simulink model "mmr_air_alternat"  (R2019a)
settings: Solver=ode4  StartTime=0.0  StopTime=ta  RelTol=1e-1
values from neighbouring files (symbols this model uses):
  g = -9.81    [MMR.m]    (also in MMR_alfa0.m; MMR_alone.m; MMR_hop_zero.m = 9.81)
  Lcol = 0.70    (= 0.7)    [MMR.m]    (also in MMR_alone.m)
  Lhk = 0.28    [MMR.m]    (also in MMR_alfa0.m; MMR_alone.m; MMR_hop_zero.m)
  Lkf = 0.28    [MMR.m]    (also in MMR_alfa0.m; MMR_alone.m; MMR_hop_zero.m)
  m = 3    [MMR.m]    (also in MMR_alfa0.m; MMR_alone.m; MMR_hop_zero.m)
  M = 15    [MMR.m]    (also in MMR_alfa0.m; MMR_alone.m; MMR_hop_zero.m)
  vxfinal = vx( length(vx) )    [MMR.m]    (also in MMR_alfa0.m; MMR_alone.m)
  vxMfinal = vxM( length(vxM) )    [MMR.m]    (also in MMR_alfa0.m; MMR_alone.m)
  vyfinal = vy( length(vy) )    [MMR.m]    (also in MMR_alfa0.m; MMR_alone.m; MMR_hop_zero.m)
  vyMfinal = vyM( length(vyM) )    [MMR.m]    (also in MMR_alfa0.m; MMR_alone.m)
  xfinal = x( length(x) )    [MMR.m]    (also in MMR_alfa0.m; MMR_alone.m)
  xMfinal = xM( length(xM) )    [MMR.m]    (also in MMR_alfa0.m; MMR_alone.m)
  yfinal = y( length(y) )    [MMR.m]    (also in MMR_alfa0.m; MMR_alone.m; MMR_hop_zero.m)
  yMfinal = yM( length(yM) )    [MMR.m]    (also in MMR_alfa0.m; MMR_alone.m)
undefined symbols (not defined in the file or in its folder): magnitude
settings Model: Creator=Jesus  LastModifiedBy=Jesus

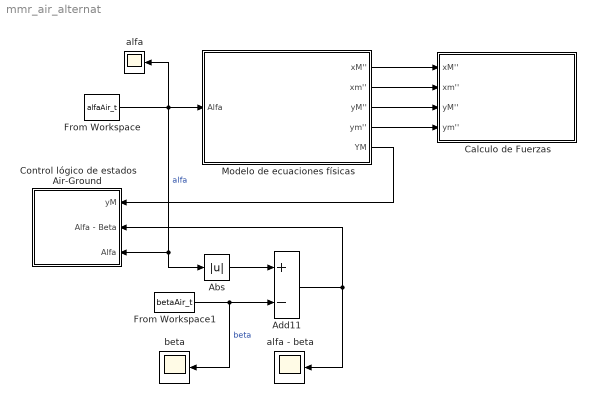
== system mmr_air_alternat ==
  Abs : Abs
  Add11 : Sum  Inputs=+-
  Calculo de Fuerzas : Subsystem
  Control lógico de estados Air-Ground : Subsystem
  From Workspace : FromWorkspace  VariableName=alfaAir_t  SampleTime=0
  From Workspace1 : FromWorkspace  VariableName=betaAir_t  SampleTime=0
  Modelo de ecuaciones físicas : Subsystem
  alfa : Scope
  alfa - beta : Scope
  beta : Scope
  wires:
  From Workspace/1 -> alfa/1, Control lógico de estados Air-Ground/3(Alfa), Abs/1, Modelo de ecuaciones físicas/1(Alfa)  "alfa"
  Add11/1 -> Control lógico de estados Air-Ground/2(Alfa - Beta), alfa - beta/1
  From Workspace1/1 -> beta/1, Add11/2  "beta"
  Modelo de ecuaciones físicas/1(xM'') -> Calculo de Fuerzas/1(xM'')
  Modelo de ecuaciones físicas/2(xm'') -> Calculo de Fuerzas/2(xm'')
  Modelo de ecuaciones físicas/3(yM'') -> Calculo de Fuerzas/3(yM'')
  Modelo de ecuaciones físicas/4(ym'') -> Calculo de Fuerzas/4(ym'')
  Modelo de ecuaciones físicas/5(YM) -> Control lógico de estados Air-Ground/1(yM)
  Abs/1 -> Add11/1

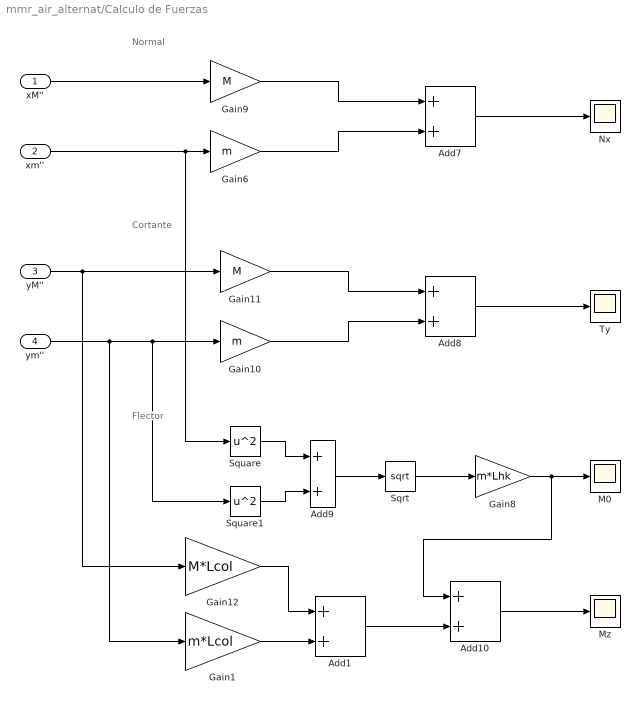
== system mmr_air_alternat/Calculo de Fuerzas ==
  note: Normal
  note: Cortante
  note: Flector
  xM'' : Inport
  xm'' : Inport  Port=2
  yM'' : Inport  Port=3
  ym'' : Inport  Port=4
  Add{1,7..10} (5 alike) : Sum
  Gain1 : Gain  Gain=m*Lcol
  Gain10 : Gain  Gain=m
  Gain11 : Gain  Gain=M
  Gain12 : Gain  Gain=M*Lcol
  Gain6 : Gain  Gain=m
  Gain8 : Gain  Gain=m*Lhk
  Gain9 : Gain  Gain=M
  M0 : Scope
  Mz : Scope
  Nx : Scope
  Sqrt : Sqrt  SaturateOnIntegerOverflow=on
  Square : Math  Operator=square  SaturateOnIntegerOverflow=on
  Square1 : Math  Operator=square  SaturateOnIntegerOverflow=on
  Ty : Scope
  wires:
  Gain10/1 -> Add8/2
  Sqrt/1 -> Gain8/1
  yM''/1 -> Gain11/1, Gain12/1
  ym''/1 -> Square1/1, Gain10/1, Gain1/1
  Square/1 -> Add9/1
  Add7/1 -> Nx/1
  Gain8/1 -> Add10/1, M0/1
  Gain6/1 -> Add7/2
  Gain11/1 -> Add8/1
  xm''/1 -> Square/1, Gain6/1
  Add9/1 -> Sqrt/1
  Add8/1 -> Ty/1
  Gain9/1 -> Add7/1
  Square1/1 -> Add9/2
  Add10/1 -> Mz/1
  xM''/1 -> Gain9/1
  Add1/1 -> Add10/2
  Gain12/1 -> Add1/1
  Gain1/1 -> Add1/2

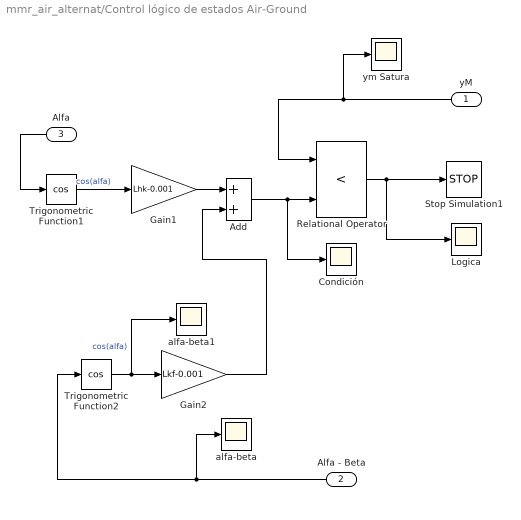
== system mmr_air_alternat/Control lógico de estados Air-Ground ==
  yM : Inport
  Alfa - Beta : Inport  Port=2
  Alfa : Inport  Port=3
  Add : Sum
  Condición : Scope
  Gain1 : Gain  Gain=Lhk-0.001
  Gain2 : Gain  Gain=Lkf-0.001
  Logica : Scope
  Relational Operator : RelationalOperator  Operator=<  OutDataTypeStr=boolean  RndMeth=Simplest
  Stop Simulation1 : Stop
  Trigonometric Function1 : Trigonometry  Operator=cos
  Trigonometric Function2 : Trigonometry  Operator=cos
  alfa-beta : Scope
  alfa-beta1 : Scope
  ym Satura : Scope
  wires:
  Relational Operator/1 -> Stop Simulation1/1, Logica/1
  Gain2/1 -> Add/2
  yM/1 -> Relational Operator/1, ym Satura/1
  Trigonometric Function2/1 -> alfa-beta1/1, Gain2/1  "cos(alfa)"
  Alfa - Beta/1 -> alfa-beta/1, Trigonometric Function2/1
  Add/1 -> Condición/1, Relational Operator/2
  Trigonometric Function1/1 -> Gain1/1  "cos(alfa)"
  Gain1/1 -> Add/1
  Alfa/1 -> Trigonometric Function1/1

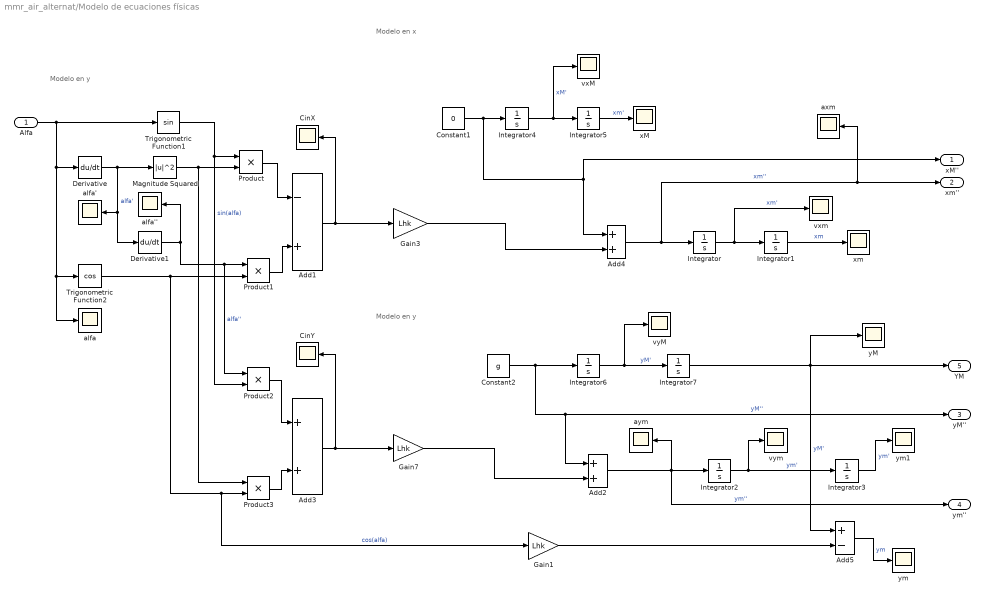
== system mmr_air_alternat/Modelo de ecuaciones físicas ==
  note: Modelo en x
  note: Modelo en y
  note: Modelo en y
  Alfa : Inport
  Add1 : Sum  Inputs=-+
  Add2 : Sum
  Add3 : Sum
  Add4 : Sum
  Add5 : Sum  Inputs=+-
  CinX : Scope
  CinY : Scope
  Constant1 : Constant  Value=0
  Constant2 : Constant  Value=g
  Derivative : Derivative  CoefficientInTFapproximation=10000
  Derivative1 : Derivative  CoefficientInTFapproximation=10000
  Gain1 : Gain  Gain=Lhk
  Gain3 : Gain  Gain=Lhk
  Gain7 : Gain  Gain=Lhk
  Integrator : Integrator  InitialCondition=vxfinal
  Integrator1 : Integrator  InitialCondition=xfinal
  Integrator2 : Integrator  InitialCondition=vyfinal
  Integrator3 : Integrator  InitialCondition=yfinal
  Integrator4 : Integrator  InitialCondition=vxMfinal
  Integrator5 : Integrator  InitialCondition=xMfinal
  Integrator6 : Integrator  InitialCondition=vyMfinal
  Integrator7 : Integrator  InitialCondition=yMfinal
  Magnitude Squared : Math  Operator=magnitude^2  SaturateOnIntegerOverflow=on
  Product{,1..3} (4 alike) : Product
  Trigonometric Function1 : Trigonometry
  Trigonometric Function2 : Trigonometry  Operator=cos
  alfa : Scope
  alfa' : Scope
  alfa'' : Scope
  axm : Scope
  aym : Scope
  vxM : Scope
  vxm : Scope
  vyM : Scope
  vym : Scope
  xM : Scope
  xm : Scope
  yM : Scope
  ym : Scope
  ym1 : Scope
  xM'' : Outport
  xm'' : Outport  Port=2
  yM'' : Outport  Port=3
  ym'' : Outport  Port=4
  YM : Outport  Port=5
  wires:
  Trigonometric Function2/1 -> Gain1/1, Product3/2, Product1/2  "cos(alfa)"
  Integrator5/1 -> xM/1  "xm'"
  Add1/1 -> Gain3/1, CinX/1
  Add5/1 -> ym/1  "ym"
  Product2/1 -> Add3/1
  Integrator1/1 -> xm/1  "xm"
  Product/1 -> Add1/1
  Add2/1 -> ym''/1, Integrator2/1, aym/1  "ym''"
  Integrator4/1 -> Integrator5/1, vxM/1  "xM'"
  Alfa/1 -> alfa/1, Trigonometric Function2/1, Derivative/1, Trigonometric Function1/1
  Derivative/1 -> alfa'/1, Derivative1/1, Magnitude Squared/1  "alfa'"
  Gain3/1 -> Add4/2
  Add4/1 -> axm/1, xm''/1, Integrator/1  "xm''"
  Product3/1 -> Add3/2
  Add3/1 -> CinY/1, Gain7/1
  Magnitude Squared/1 -> Product/2, Product3/1
  Integrator2/1 -> Integrator3/1, vym/1  "ym'"
  Integrator/1 -> vxm/1, Integrator1/1  "xm'"
  Product1/1 -> Add1/2
  Gain7/1 -> Add2/2
  Integrator6/1 -> Integrator7/1, vyM/1  "yM'"
  Constant2/1 -> yM''/1, Add2/1, Integrator6/1  "yM''"
  Derivative1/1 -> alfa''/1, Product1/1, Product2/1  "alfa''"
  Trigonometric Function1/1 -> Product2/2, Product/1  "sin(alfa)"
  Constant1/1 -> Integrator4/1, Add4/1, xM''/1
  Integrator7/1 -> YM/1, Add5/1, yM/1  "yM'"
  Gain1/1 -> Add5/2
  Integrator3/1 -> ym1/1  "ym'"
